simulink model "actuatorsC172p"  (R2026a)
settings: configuration reference "standardSILConfiguraitonParams" (kept outside this file)
undefined symbols (not defined in the file or in its folder): aileronDeflRateLimit_degps, elevatorDeflRateLimit_degps, maxAilDefl_deg, maxElevatorDefl_deg, maxRudderDefl_deg, rudderDeflRateLimit_degps, ServosF16Bus, tauAilerons_s, tauElevator_s, tauRudder_s
settings Model: Creator=GTAR  LastModifiedBy=Edison Altamirano
settings ConfigSetRef: SourceName=standardSILConfiguraitonParams  SourceLocation=Base Workspace

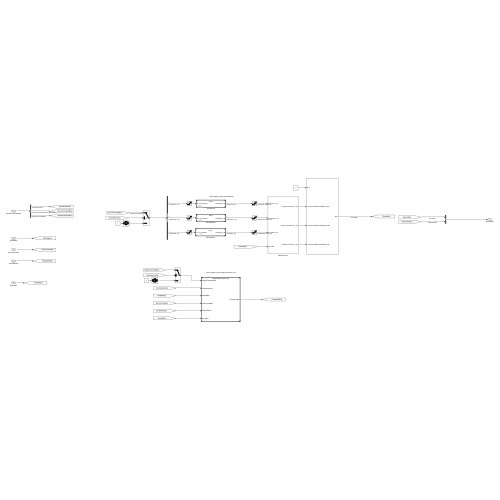
[thumbnail: Simulink's stored preview of the top-level diagram]
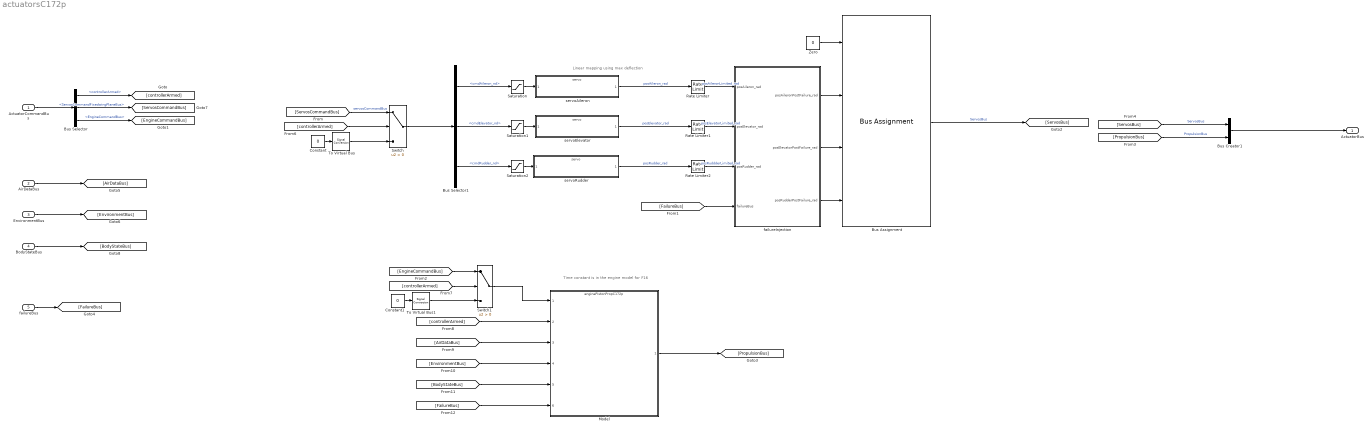
== system actuatorsC172p ==
  note: Linear mapping using max deflection
  note: Time constant is in the engine model for F16
  ActuatorCommandBus : Inport  OutDataTypeStr=Bus: ActuatorCommandBus
  AirDataBus : Inport  Port=2  OutDataTypeStr=Bus: AirDataBus
  EnvironmentBus : Inport  Port=3  OutDataTypeStr=Bus: EnvironmentBus
  BodyStateBus : Inport  Port=4  OutDataTypeStr=Bus: BodyStateBus
  failureBus : Inport  Port=5  OutDataTypeStr=Bus: FailureBus
  Bus Assignment : BusAssignment  AssignedSignals=ServosF16Bus.posAileron_rad,ServosF16Bus.posElevator_rad,ServosF16Bus.posRudder_rad
  Bus Creator1 : BusCreator  Inputs=2  OutDataTypeStr=Bus: ActuatorBus
  Bus Selector : BusSelector  OutputSignals=controllerArmed,ServosCommandBus.ServosCommandFixedwingPlaneBus,EngineCommandBus
  Bus Selector1 : BusSelector  OutputSignals=cmdAileron_nd,cmdElevator_nd,cmdRudder_nd
  Constant : Constant  Value=0  VectorParams1D=off  OutDataTypeStr=Bus: ServosCommandFixedwingPlaneBus  SampleTime=-1
  Constant1 : Constant  Value=0  OutDataTypeStr=Bus: EngineCommandBus
  Model : ModelReference  ModelNameDialog=enginePistonPropC172p.slx  SimulationMode=Normal  ModelReferenceVersion=1.4
  Rate Limiter : RateLimiter  RisingSlewLimit=deg2rad(aileronDeflRateLimit_degps)  FallingSlewLimit=-deg2rad(aileronDeflRateLimit_degps)  SampleTimeMode=inherited
  Rate Limiter1 : RateLimiter  RisingSlewLimit=deg2rad(elevatorDeflRateLimit_degps)  FallingSlewLimit=-deg2rad(elevatorDeflRateLimit_degps)  SampleTimeMode=inherited
  Rate Limiter2 : RateLimiter  RisingSlewLimit=deg2rad(rudderDeflRateLimit_degps)  FallingSlewLimit=deg2rad(-rudderDeflRateLimit_degps)  SampleTimeMode=inherited
  Saturation : Saturate  UpperLimit=1  LowerLimit=-1
  Saturation1 : Saturate  UpperLimit=1  LowerLimit=-1
  Saturation2 : Saturate  UpperLimit=1  LowerLimit=-1
  Switch : Switch  Criteria=u2 > Threshold  SaturateOnIntegerOverflow=off  InputSameDT=off
  Switch1 : Switch  Criteria=u2 > Threshold  SaturateOnIntegerOverflow=off  InputSameDT=off
  To Virtual Bus : SignalConversion  ConversionOutput=Virtual bus  OverrideOpt=off
  To Virtual Bus1 : SignalConversion  ConversionOutput=Virtual bus  OverrideOpt=off
  Zero : Constant  Value=0  OutDataTypeStr=Bus: ServosBus
  failureInjection : Subsystem
  servoAileron : ModelReference  ModelNameDialog=servo.slx  UsingDefaultArgumentValue=0,0,0  SimulationMode=Normal  ModelReferenceVersion=1.21  scale=deg2rad(maxAilDefl_deg)  tfNumerator=1  tfDenominator=[tauAilerons_s 1]
  servoElevator : ModelReference  ModelNameDialog=servo.slx  UsingDefaultArgumentValue=0,0,0  SimulationMode=Normal  ModelReferenceVersion=1.21  scale=deg2rad(maxElevatorDefl_deg)  tfNumerator=1  tfDenominator=[tauElevator_s 1]
  servoRudder : ModelReference  ModelNameDialog=servo.slx  UsingDefaultArgumentValue=0,0,0  SimulationMode=Normal  ModelReferenceVersion=1.21  scale=deg2rad(maxRudderDefl_deg)  tfNumerator=1  tfDenominator=[tauRudder_s 1]
  ActuatorBus : Outport  OutDataTypeStr=Bus: ActuatorBus
  wires:
  Bus Assignment/1 -> [ServosBus]  "ServosBus"
  Model/1 -> [PropulsionBus]
  [PropulsionBus] -> Bus Creator1/2  "PropulsionBus"
  [ServosBus] -> Bus Creator1/1  "ServosBus"
  Bus Selector1/1 -> Saturation/1  "<cmdAileron_nd>"
  Bus Selector1/2 -> Saturation1/1  "<cmdElevator_nd>"
  Bus Selector1/3 -> Saturation2/1  "<cmdRudder_nd>"
  Bus Creator1/1 -> ActuatorBus/1
  [ServosCommandBus] -> Switch/1  "servosCommandBus"
  Switch/1 -> Bus Selector1/1
  [controllerArmed] -> Switch/2
  Constant/1 -> To Virtual Bus/1
  Switch1/1 -> Model/1
  Constant1/1 -> To Virtual Bus1/1
  [controllerArmed] -> Switch1/2
  To Virtual Bus/1 -> Switch/3
  To Virtual Bus1/1 -> Switch1/3
  AirDataBus/1 -> [AirDataBus]
  [AirDataBus] -> Model/3
  EnvironmentBus/1 -> [EnvironmentBus]
  [EnvironmentBus] -> Model/4
  BodyStateBus/1 -> [BodyStateBus]
  [BodyStateBus] -> Model/5
  [controllerArmed] -> Model/2
  ActuatorCommandBus/1 -> Bus Selector/1
  Bus Selector/1 -> [controllerArmed]  "<controllerArmed>"
  Bus Selector/2 -> [ServosCommandBus]  "<ServosCommandFixedwingPlaneBus>"
  Bus Selector/3 -> [EngineCommandBus]  "<EngineCommandBus>"
  Zero/1 -> Bus Assignment/1
  servoElevator/1 -> Rate Limiter1/1  "posElevator_rad"
  servoRudder/1 -> Rate Limiter2/1  "posRudder_rad"
  servoAileron/1 -> Rate Limiter/1  "posAileron_rad"
  [EngineCommandBus] -> Switch1/1
  Saturation2/1 -> servoRudder/1
  Saturation1/1 -> servoElevator/1
  Saturation/1 -> servoAileron/1
  Rate Limiter/1 -> failureInjection/1(posAileron_rad)  "posAileronLimited_rad"
  Rate Limiter1/1 -> failureInjection/2(posElevator_rad)  "posElevatorLimited_rad"
  Rate Limiter2/1 -> failureInjection/3(posRudder_rad)  "posRuddderLimited_rad"
  [FailureBus] -> failureInjection/4(failureBus)
  failureInjection/1(posAileronPostFailure_rad) -> Bus Assignment/2
  failureInjection/2(posElevatorPostFailure_rad) -> Bus Assignment/3
  failureInjection/3(posRudderPostFailure_rad) -> Bus Assignment/4
  [FailureBus] -> Model/6
  failureBus/1 -> [FailureBus]

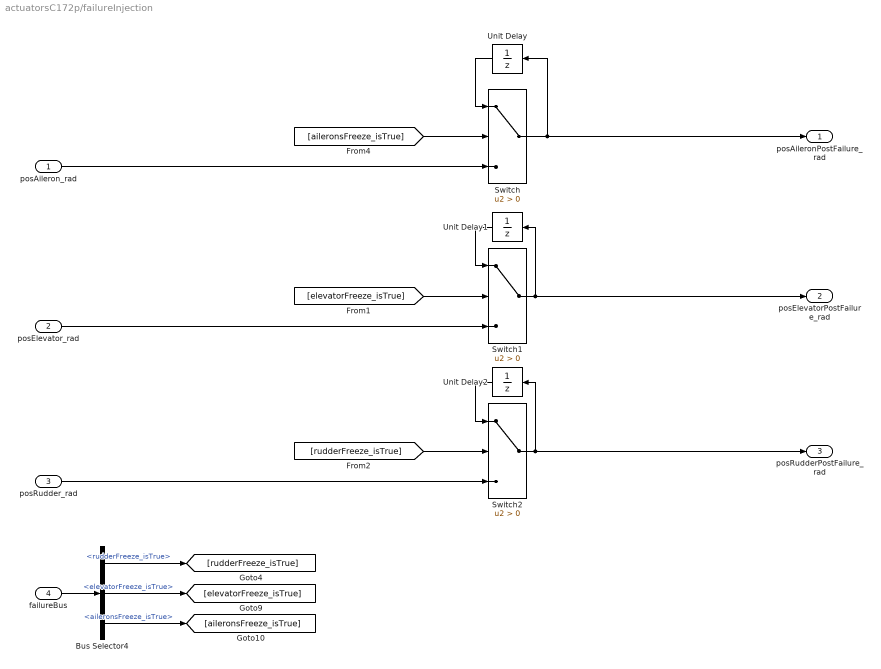
== system actuatorsC172p/failureInjection ==
  posAileron_rad : Inport
  posElevator_rad : Inport  Port=2
  posRudder_rad : Inport  Port=3
  failureBus : Inport  Port=4
  Bus Selector4 : BusSelector  OutputSignals=rudderFreeze_isTrue,elevatorFreeze_isTrue,aileronsFreeze_isTrue
  Switch : Switch  Criteria=u2 > Threshold  SaturateOnIntegerOverflow=off  InputSameDT=off
  Switch1 : Switch  Criteria=u2 > Threshold  SaturateOnIntegerOverflow=off  InputSameDT=off
  Switch2 : Switch  Criteria=u2 > Threshold  SaturateOnIntegerOverflow=off  InputSameDT=off
  Unit Delay : UnitDelay  SampleTime=-1
  Unit Delay1 : UnitDelay  SampleTime=-1
  Unit Delay2 : UnitDelay  SampleTime=-1
  posAileronPostFailure_rad : Outport
  posElevatorPostFailure_rad : Outport  Port=2
  posRudderPostFailure_rad : Outport  Port=3
  wires:
  [aileronsFreeze_isTrue] -> Switch/2
  posAileron_rad/1 -> Switch/3
  Switch/1 -> posAileronPostFailure_rad/1, Unit Delay/1
  Unit Delay/1 -> Switch/1
  posElevator_rad/1 -> Switch1/3
  [elevatorFreeze_isTrue] -> Switch1/2
  posRudder_rad/1 -> Switch2/3
  [rudderFreeze_isTrue] -> Switch2/2
  Switch1/1 -> posElevatorPostFailure_rad/1, Unit Delay1/1
  Unit Delay1/1 -> Switch1/1
  Switch2/1 -> posRudderPostFailure_rad/1, Unit Delay2/1
  Unit Delay2/1 -> Switch2/1
  Bus Selector4/2 -> [elevatorFreeze_isTrue]  "<elevatorFreeze_isTrue>"
  Bus Selector4/3 -> [aileronsFreeze_isTrue]  "<aileronsFreeze_isTrue>"
  Bus Selector4/1 -> [rudderFreeze_isTrue]  "<rudderFreeze_isTrue>"
  failureBus/1 -> Bus Selector4/1
